simulink model "ASK"  (Simulink 7.2)
settings: Solver=ode45  StartTime=0.0  StopTime=100  RelTol=1e-3
libraries: commrandsrc2 x1, dsparch4 x1
settings Model: Creator=usuario  LastModifiedBy=USUARIO
settings OptimizationCC: InlineInvariantSignals=on  InitFltsAndDblsToZero=on
settings DebuggingCC: SaveWithParameterizedLinksMsg=none  SignalResolutionControl=TryResolveAllWithWarning  MultiTaskDSMMsg=warning  MultiTaskCondExecSysMsg=none  StrictBusMsg=None
settings RTWCC: IncludeERTFirstTime=on
settings GRTTargetCC: TargetFcnLib=ansi_tfl_tmw.mat

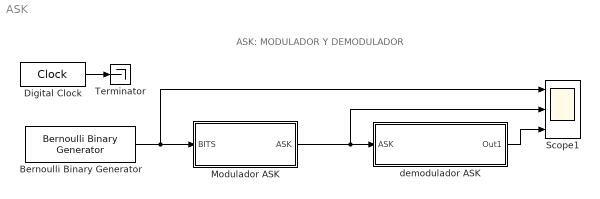
== system ASK ==
  note: ASK: MODULADOR Y DEMODULADOR
  Bernoulli Binary Generator : commrandsrc2/Bernoulli Binary Generator  DialogController=commDDGCreate  DialogControllerArgs=DataTag0  SystemSampleTime=-1  P=0.4  seed=81  Ts=5  frameBased=off  sampPerFrame=1  orient=off  outDataType=double
  Digital Clock : DigitalClock  SampleTime=0.001
  Modulador ASK : Subsystem
  Scope1 : Scope  NumInputPorts=3
      settings: YMin=-5~-5~-5  YMax=5~5~5  SaveName=ScopeData3
  Terminator : Terminator
  demodulador ASK : Subsystem
  wires:
  Bernoulli Binary Generator/1 -> Modulador ASK/1(BITS), Scope1/1
  Modulador ASK/1(ASK) -> demodulador ASK/1(ASK), Scope1/2
  demodulador ASK/1(Out1) -> Scope1/3
  Digital Clock/1 -> Terminator/1

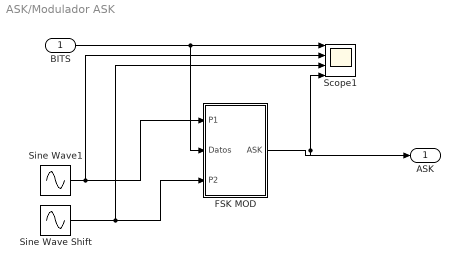
== system ASK/Modulador ASK ==
  BITS : Inport  OutDataType=sfix(16)  OutScaling=2^0
  FSK MOD : Subsystem
  Scope1 : Scope  NumInputPorts=4
      settings: YMin=-2~-3~-3~-3  YMax=2~3~3~3
  Sine Wave Shift : Sin  SineType=Sample based  Amplitude=0.5  Frequency=2*10*pi  Phase=-pi  Samples=50  SampleTime=1/20
  Sine Wave1 : Sin  SineType=Sample based  Amplitude=2  Frequency=2*10*pi  Samples=50  SampleTime=1/20
  ASK : Outport  OutDataType=sfix(16)  OutScaling=2^0
  wires:
  BITS/1 -> Scope1/1, FSK MOD/2(Datos)
  Sine Wave1/1 -> Scope1/2, FSK MOD/1(P1)
  Sine Wave Shift/1 -> Scope1/3, FSK MOD/3(P2)
  FSK MOD/1(ASK) -> Scope1/4, ASK/1

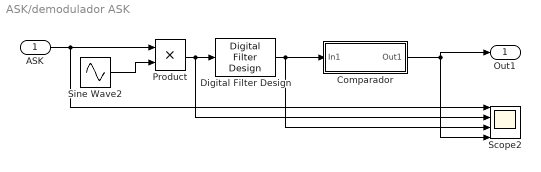
== system ASK/demodulador ASK ==
  ASK : Inport  OutDataType=sfix(16)  OutScaling=2^0
  Comparador : Subsystem
  Digital Filter Design : dsparch4/Digital Filter Design  SystemSampleTime=-1  mwdsp_browser_bugfix_var=off
  Product : Product  OutDataType=sfix(16)  OutScaling=2^0  RndMeth=Zero
  Scope2 : Scope  NumInputPorts=4
      settings: YMin=-2~-3~-3~-5  YMax=2~3~3~5
  Sine Wave2 : Sin  SineType=Sample based  Frequency=2*10*pi  Samples=50  SampleTime=1/20
  Out1 : Outport  OutDataType=sfix(16)  OutScaling=2^0
  wires:
  ASK/1 -> Scope2/1, Product/1
  Sine Wave2/1 -> Product/2
  Product/1 -> Digital Filter Design/1, Scope2/2
  Digital Filter Design/1 -> Scope2/3, Comparador/1(In1)
  Comparador/1(Out1) -> Scope2/4, Out1/1

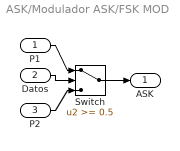
== system ASK/Modulador ASK/FSK MOD ==
  P1 : Inport  OutDataType=sfix(16)  OutScaling=2^0
  Datos : Inport  Port=2  OutDataType=sfix(16)  OutScaling=2^0
  P2 : Inport  Port=3  OutDataType=sfix(16)  OutScaling=2^0
  Switch : Switch  Threshold=0.5
  ASK : Outport  OutDataType=sfix(16)  OutScaling=2^0
  wires:
  P1/1 -> Switch/1
  Datos/1 -> Switch/2
  Switch/1 -> ASK/1
  P2/1 -> Switch/3

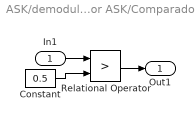
== system ASK/demodulador ASK/Comparador ==
  In1 : Inport  OutDataType=sfix(16)  OutScaling=2^0
  Constant : Constant  Value=0.5  OutDataType=sfix(16)  OutScaling=2^0
  Relational Operator : RelationalOperator  Operator=>  LogicOutDataTypeMode=boolean  OutDataTypeStr=boolean
  Out1 : Outport  OutDataType=sfix(16)  OutScaling=2^0
  wires:
  Constant/1 -> Relational Operator/2
  In1/1 -> Relational Operator/1
  Relational Operator/1 -> Out1/1
